simulink library "xps_library"  (Simulink 7.3)
settings: Solver=ode45  SolverMode=SingleTasking  StartTime=0.0  StopTime=10.0  RelTol=1e-3
undefined symbols (not defined in the file): powerpc405, sys_clk, xps_library_software_register_user_data_in
libraries: xbsIndex_r4 x699, simulink x61, casper_library x50, dspsigops x48, xps_library x20, xbsIndex_r3 x2
(part 1 of 9)
settings Model: Creator=hchen05  LastModifiedBy=arccadmin

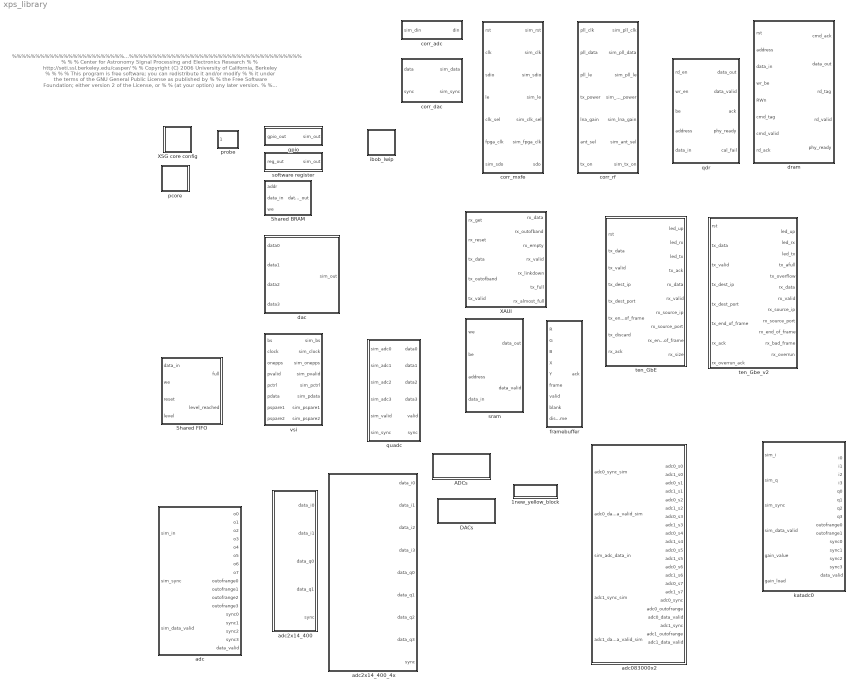
== system xps_library ==
  note: %%%%%%%%%%%%%%%%%%%%%%%%%%%%%%%%%%%%%%%%%%%%%%%%%%%%%%%%%%%%%%%%%%%%%%%%%%%%%%%
      | %                                                                             %
      | %   Center for Astronomy Signal Processing and Electronics Research           %
      | %   http://seti.ssl.berkeley.edu/casper/                                      %
      | %   Copyright (C) 2006 University of California, Berkeley                     %
      | %                                                                             %
      | %   This program is free software; you can redistribute it and/or modify      %
      | %   it under the terms of the GNU General Public License as published by      %
      | %   the Free Software Foundation; either version 2 of the License, or         %
      | %   (at your option) any later version.                                       %
      | %                                                                             %
      | %   This program is distributed in the hope that it will be useful,           %
      | %   but WITHOUT ANY WARRANTY; without even the implied warranty of            %
      | %   MERCHANTABILITY or FITNESS FOR A PARTICULAR PURPOSE.  See the             %
      | %   GNU General Public License for more details.                              %
      | %                                                                             %
      | %   You should have received a copy of the GNU General Public License along   %
      | %   with this program; if not, write to the Free Software Foundation, Inc.,   %
      | %   51 Franklin Street, Fifth Floor, Boston, MA 02110-1301 USA.               %
      | %                                                                             %
      | %%%%%%%%%%%%%%%%%%%%%%%%%%%%%%%%%%%%%%%%%%%%%%%%%%%%%%%%%%%%%%%%%%%%%%%%%%%%%%%
  1new_yellow_block : Subsystem  Tag=xps:block_name
  ADCs : Subsystem
  DACs : Subsystem
  Shared BRAM : Subsystem  Tag=xps:bram  mask{arith_type=Signed  (2's comp), addr_width=11, data_width=32, data_bin_pt=0, init_vals=[1:2^11], sample_rate=1}
      mask prompts: arith_type "Output Data Type"; addr_width "Address width"; data_width "Data Width"; data_bin_pt "Data Binary Point"; init_vals "Initial values (simulation only)"; sample_rate "Sample rate"
      mask init:
      | shared_bram_mask;
      mask StyleString: popup(Unsigned|Signed  (2's comp)),edit,edit,edit,edit,edit
  Shared FIFO : Subsystem  Tag=xps:fifo  mask{io_dir=To Processor, arith_type=Unsigned, data_width=32, data_bin_pt=0, fifo_length=512}
      mask prompts: io_dir "I/O Direction:"; arith_type "Data Type:"; data_width "Data Width:"; data_bin_pt "Data Binary Point:"; fifo_length "Depth:"
      mask init:
      | fifo_mask;
      mask StyleString: popup(From Processor|To Processor),popup(Unsigned|Signed  (2's comp)),popup(4|8|16|32|64|128|256),edit,popup(512|1024|2048|4096|8192|16384|32768|65536)
  XAUI : Subsystem  Tag=xps:xaui  mask(xaui){demux=1, port=ROACH:0, open_phy=on, show_param=off, pre_emph=3, swing=800}
      mask prompts: open_phy "Use KAT open PHY"; show_param "---------------------- Show Implementation Parameters -----------------------------------------------------------------------------------"; pre_emph "Pre-emphasis"; swing "Differential swing"
      mask help: XAUI block for sending and receiving point-to-point, streaming data over the BEE2 and iBOB's CX4 connectors. NOTE: A new version of this block is in development.
      mask init:
      | xaui_mask;
      mask Help: eval('xlWeb([getenv(''MLIB_ROOT''), ''\doc\html\com_xaui\com_xaui.html''])')
      mask StyleString: popup(1|2),popup(iBOB:0|iBOB:1|BEE2_ctrl:0|BEE2_ctrl:1|BEE2_usr:0|BEE2_usr:1|BEE2_usr:2|BEE2_usr:3|CORR:0|ROACH:0|ROACH:1|ROACH:2|ROACH:3),checkbox,checkbox,popup(0|1|2|3),popup(400|500|600|700|800)
      mask CallbackString:
      | |||myname=gcb;
      | if strcmp(get_param(myname, 'show_param'), 'on')
      |     set_param(myname, 'MaskVisibilities', {'on','on','on','on','on','on'});
      | else
      |     set_param(myname, 'MaskVisibilities', {'on','on','on','on','off','off'});
      | end||
  XSG core config : Subsystem  Tag=xps:xsg  mask(xsg core config){hw_sys=iBOB, ibob_linux=off, clk_src=sys_clk, iBOB_clk_src=sys_clk, BEE2_ctrl_clk_src=sys_clk, BEE2_usr_clk_src=sys_clk, ROACH_clk_src=sys_clk, CORR_clk_src=sys_clk, gpio_clk_io_group=iBOB:sma, gpio_clk_bit_index=0, clk_rate=100, sample_period=1, synthesis_tool=XST, mpc_type=powerpc405}
      mask prompts: hw_sys "Hardware Platform"; ibob_linux "Include Linux add-on board support"; clk_src "User IP Clock source"; iBOB_clk_src "User IP Clock source"; BEE2_ctrl_clk_src "User IP Clock Source"; BEE2_usr_clk_src "User IP Clock Source"; ROACH_clk_src "User IP Clock Source"; CORR_clk_src "User IP Clock Source"; gpio_clk_io_group "GPIO Clock Pin I/O group"; gpio_clk_bit_index "GPIO Clock Pin bit index"; clk_rate "User IP Clock Rate (MHz)"; sample_period "Sample Period"; synthesis_tool "Synthesis Tool:"; mpc_type "Processor:"
      mask help:
      | The XSG Core Config block is used to configure the System Generator design
      | for the bee_xps toolflow. Settings here are used to configure the
      | Xilinx System Generator block parameters automatically, and control toolflow
      | script  execution. It needs to be at the top level of all designs being compiled
      | with the bee_xps toolflow.
      mask init:
      | xps_xsg_conf_mask;
      mask Help: eval('xlWeb([getenv(''MLIB_ROOT''), ''\doc\html\sys_xsg_core_config\sys_xsg_core_config.html''])')
      mask StyleString: popup(iBOB|BEE2_ctrl|BEE2_usr|ROACH:sx95t|ROACH:lx110t|CORR),checkbox,edit,popup(sys_clk|sys_clk2x|usr_clk|usr_clk2x|adc0_clk|adc1_clk|dac0_clk|dac1_clk),popup(sys_clk|sys_clk2x|usr_clk|usr_clk2x),popup(sys_clk|sys_clk2x|usr_clk|usr_clk2x),popup(sys_clk|sys_clk2x|arb_clk|aux0_clk|aux0_clk2x|aux1_clk|aux1_clk2x|adc0_clk|adc1_clk|dac0_clk|dac1_clk),popup(sys_clk|sys_clk2x|usr_clk|usr_clk2x),popup(iBOB:gpio0|iBOB:gpio1|iBOB:gpio2|iBOB:gpio3|iBOB:sma|iBOB:zdok0|iBOB:zdok1|iBOB:mdr),edit,edit,edit,popup(Leonardo Spectrum|Synplify|Synplify Pro|XST),edit
      mask CallbackString: xps_xsg_conf_callback;|||xps_xsg_conf_callback;|xps_xsg_conf_callback;|xps_xsg_conf_callback;|xps_xsg_conf_callback;|xps_xsg_conf_callback;||||||
      mask Display: fprintf(['MSSGE\n', hw_sys]);
  adc : Subsystem  Tag=xps:adc  mask(adc){adc_brd=adc0, adc_clk_rate=800, adc_interleave=on, sample_period=1}
      mask prompts: adc_brd "ADC board"; adc_clk_rate "ADC clock rate (MHz)"; adc_interleave "ADC interleave mode"; sample_period "Sample period"
      mask help: The ADC block converts analog inputs to digital outputs. Every clock cycle, the inputs are sampled and digitized to 8 bit binary point numbers in the range of [-1, 1) and are then output by the adc.
      mask init:
      | adc_mask;
      mask Help: eval('xlWeb([getenv(''MLIB_ROOT''), ''\doc\html\sys_adc\sys_adc.html''])')
      mask StyleString: popup(adc0|adc1),edit,checkbox,edit
  adc083000x2 : Subsystem  Tag=xps:adc083000x2  mask(adc_083000x2){use_adc0=on, use_adc1=on, demux_adc=off, clock_sync=on, verbose=off, using_ctrl=on, adc_clk_rate=1000, sample_period=1, bit_width=8}
      mask prompts: use_adc0 "Use ZD0K0?"; use_adc1 "Use ZDOK1?"; demux_adc "Demux ADCs by 2?"; clock_sync "Interleave 2 ADC boards?"; verbose "Verbose Block Creation?"; using_ctrl "Add ports for control registers?"; adc_clk_rate "ADC clock rate (MHz)"; sample_period "Sample Period"; bit_width "Output Bit Width"
      mask help:
      | The ADC block converts analog inputs to digital outputs.
      | Every clock cycle, the inputs are sampled and digitized to
      | 8 bit binary point numbers in the range of [-1, 1).
      |
      | Online block-specific documentation: http://casper.berkeley.edu/wiki/Adc083000
      mask init:
      | adc083000_mask;
      mask Help: eval('xlWeb([getenv(''MLIB_ROOT''), ''\doc\html\sys_adc\sys_adc.html''])')
  adc2x14_400 : Subsystem  Tag=xps:adc2x14_400  mask(ADC board 2xADS5474 Interface Block){adc_brd=0, adc_clk_rate=400}
      mask prompts: adc_brd "ADC Board"; adc_clk_rate "ADC Clock Rate (MHz)"
      mask help: Interface block for the MKID 14-bits 400 MHz ADC board (2xADS5474).
      mask init:
      | adc2x14_400_mask;
      mask StyleString: popup(0|1),edit
  adc2x14_400_4x : Subsystem  Tag=xps:adc2x14_400_4x  mask(2x 14-400 ADC Interface Block){adc_brd=1, adc_clk_rate=400}
      mask prompts: adc_brd "ADC Board"; adc_clk_rate "ADC Clock Rate (MHz)"
      mask help: Interface block for the 14-bits 400 MHz DC board (2xADS5474).
      mask init:
      | adc2x14_400_4x_mask;
      mask StyleString: popup(0|1),edit
  corr_adc : Subsystem  Tag=xps:corr_adc  mask{adc_brd=CORR:adc_i, arith_type=Signed  (2's comp), data_bin_pt=11, reg_clk_phase=0, sample_period=1}
      mask prompts: adc_brd "ADC:"; arith_type "Data type:"; data_bin_pt "Binary point:"; reg_clk_phase "Input sample clock phase:"; sample_period "Sample period:"
      mask init:
      | corr_adc_mask;
      mask StyleString: popup(CORR:adc_i|CORR:adc_q),popup(Unsigned|Signed  (2's comp)),edit,popup(0|90|180|270),edit
  corr_dac : Subsystem  Tag=xps:corr_dac  mask{arith_type=Unsigned, bin_pt=12, reg_clk_phase=0, sample_period=1}
      mask prompts: arith_type "Data Type:"; bin_pt "Data binary point (14-bit data):"; reg_clk_phase "Output sample clock phase:"; sample_period "Sample period:"
      mask init:
      | corr_dac_mask;
      mask StyleString: popup(Boolean|Unsigned|Signed  (2's comp)),edit,popup(0|90|180|270),edit
  corr_mxfe : Subsystem  Tag=xps:corr_mxfe  mask{reg_clk_phase=0, sample_period=1}
      mask prompts: reg_clk_phase "Input sample clock phase:"; sample_period "Sample period:"
      mask init:
      | corr_mxfe_mask;
      mask StyleString: popup(0|90|180|270),edit
  corr_rf : Subsystem  Tag=xps:corr_rf  mask{arith_type=Unsigned, bin_pt=0, sample_period=1}
      mask prompts: arith_type "TX power data type:"; bin_pt "TX power binary point (3-bit data):"; sample_period "Sample period:"
      mask init:
      | corr_rf_mask;
      mask StyleString: popup(Boolean|Unsigned|Signed  (2's comp)),edit,edit
  dac : Subsystem  Tag=xps:dac  mask(dac){dac_brd=iBOB:dac0, dac_clk_rate=800, sample_period=1, show_param=off, invert_clock=off}
      mask prompts: dac_brd "DAC board"; dac_clk_rate "DAC clock rate (MHz)"; sample_period "Sample period"; show_param "---------------------- Show Implementation Parameters -----------------------------------------------------------------------------------"; invert_clock "Invert output clock phase"
      mask help: Interface to SiBeam single Atmel TS86101G2B DAC board. The DAC block converts 4 digital inputs to 1 analog output. The dac runs at 4x FPGA clock frequency, outputting analog converted samples 0 through 3 each FPGA clock cycle.
      mask init:
      | dac_mask;
      mask Help: eval('xlWeb([getenv(''MLIB_ROOT''), ''\doc\html\sys_dac\sys_dac.html''])')
      mask StyleString: popup(iBOB:dac0|iBOB:dac1),edit,edit,checkbox,checkbox
      mask CallbackString:
      | |||myname=gcb;
      | if strcmp(get_param(myname, 'show_param'), 'on')
      |     set_param(myname, 'MaskVisibilities', {'on','on','on','on','on'});
      | else
      |     set_param(myname, 'MaskVisibilities', {'on','on','on','on','off'});
      | end|
  dram : Subsystem  Tag=xps:dram  mask(dram){dimm=1, arith_type=Unsigned, bin_pt=0, ip_clock=200, sample_period=1, bram_fifos=off, disable_tag=off, use_sim=off, ram_depth=18, bank_mgt=off, wide_data=off, half_burst=off, use_sniffer=off}
      mask prompts: arith_type "Data Type"; bin_pt "Data binary point"; ip_clock "Datapath clock rate (MHz)"; sample_period "Sample period"; bram_fifos "Use BRAM FIFOs"; disable_tag "Disable tag FIFO"; use_sim "Simulate DRAM using ModelSim"; ram_depth "Lesser simulation address width"; bank_mgt "Enable bank management"; wide_data "Use wide data bus (288 bits)"; half_burst "Use half-burst"; use_sniffer "Include CPU Interface"
      mask help:
      | Interface to 1GB DDR2 DIMMs on BEE2.
      |
      | To simulate using ModelSim, place a ModelSim block named 'ModelSim' (case-sensitive) in the top level of the design.
      |
      | Commands that are clocked-in are executed with an unknown delay, however, execution order is maintained.
      mask init:
      | dram_mask(gcb, use_sim, wide_data);
      mask Help: eval('xlWeb([getenv(''MLIB_ROOT''), ''\doc\html\sys_dram\sys_dram.html''])')
      mask StyleString: popup(1|2|3|4),popup(Boolean|Unsigned|Signed  (2's comp)),edit,edit,edit,checkbox,checkbox,checkbox,edit,checkbox,checkbox,checkbox,checkbox
      mask CallbackString:
      | |||||||myname=gcb;
      | if strcmp(get_param(myname, 'use_sim'), 'off')
      |     masks = get_param(myname, 'MaskEnables');
      |     masks{9} = 'on';
      |     set_param(myname, 'MaskEnables', masks);
      | else
      |     masks = get_param(myname, 'MaskEnables');
      |     masks{9} = 'off';
      |     set_param(myname, 'MaskEnables', masks);
      | end|||myname=gcb;
      | if strcmp(get_param(myname, 'wide_data'), 'off')
      |     masks = get_param(myname, 'MaskEnables');
      |     masks{12} = 'on';
      |     set_param(myname, 'MaskEnables', masks);
      | else
      |     set_param(myname, 'half_burst', 'off');
      |     masks = get_param(myname, 'MaskEnables');
      |     masks{12} = 'off';
      |     set_param(myname, 'MaskEnables', masks);
      | end||
  framebuffer : Subsystem  Tag=xps:framebuffer  mask(framebuffer){dimm=2, sample_period=1}
      mask prompts: sample_period "Sample period"
      mask help: Interface to Framebuffer.
      mask init:
      | framebuffer_mask;
      mask StyleString: popup(2|3|4),edit
  gpio : Subsystem  Tag=xps:gpio  mask(gpio){io_group=iBOB:led, io_dir=out, arith_type=Boolean, bitwidth=1, bin_pt=0, bit_index=1, sample_period=1, use_single_ended=off, use_ddr=off, reg_iob=on, reg_clk_phase=0, termination=None}
      mask prompts: io_group "I/O group"; io_dir "I/O direction"; arith_type "Data Type"; bitwidth "Data bitwidth"; bin_pt "Data binary point"; bit_index "GPIO bit index"; sample_period "Sample period"; use_single_ended "Use as single-ended"; use_ddr "Use DDR"; reg_iob "Pack register in the pad"; reg_clk_phase "Register clock phase"; termination "Termination method"
      mask help: GPIO interfaces for BEE2, iBOB, ROACH and CORR boards.
      mask init:
      | gpio_mask;
      mask StyleString: popup(iBOB:led|iBOB:dipsw|iBOB:gpio0|iBOB:gpio1|iBOB:gpio2|iBOB:gpio3|iBOB:zdok0|iBOB:zdok1|iBOB:mdr|iBOB:sma|BEE2_ctrl:led|BEE2_ctrl:downlink1|BEE2_ctrl:downlink2|BEE2_ctrl:downlink3|BEE2_ctrl:downlink4|BEE2_usr:led|BEE2_usr:bus_ctrl|BEE2_usr:bus_data|BEE2_usr:uplink|BEE2_usr:leftlink|BEE2_usr:rightlink|ROACH:led|ROACH:gpioa|ROACH:gpioa_oe_n|ROACH:gpiob|ROACH:gpiob_oe_n|ROACH:qsh|ROACH:zdok0|ROACH:zdok1|CORR:four_buttons|CORR:six_buttons|CORR:led|CORR:jumper_driver|CORR:jumper_receiver),popup(in|out),popup(Boolean|Unsigned|Signed  (2's comp)),edit,edit,edit,edit,checkbox,checkbox,checkbox,popup(0|90|180|270),popup(None|Pullup|Pulldown)
      mask CallbackString:
      | if ~isempty(find(strcmp(get_param(gcb, 'io_group'), {'iBOB:zdok0' 'iBOB:zdok1' 'iBOB:mdr' 'ROACH:qsh' 'ROACH:zdok0' 'ROACH:zdok1'})))
      |     set_param(gcb, 'MaskVisibilities', {'on','on','on','on','on','on','on','on','on','on','on','on'});
      | else
      |     set_param(gcb, 'MaskVisibilities', {'on','on','on','on','on','on','on','off','on','on','on','on'});
      | end||||||||if strcmp(get_param(gcb,'use_ddr'),'on')
      |     set_param(gcb,'reg_iob','on');
      |     set_param(gcb,'MaskEnables', {'on' 'on' 'on' 'on' 'on' 'on' 'on' 'on' 'on' 'off' 'on' 'on'});
      | else
      |     set_param(gcb,'MaskEnables', {'on' 'on' 'on' 'on' 'on' 'on' 'on' 'on' 'on' 'on' 'on' 'on'});
      | end|||
  ibob_lwip : Subsystem
      mask Type: ibobethlite
      mask Description: Attaches SRAM0 to the PLB bus and adds LWIP support.
      mask Display: fprintf('IBOB\nLWIP');
  katadc0 : Subsystem  Tag=xps:katadc  mask(adc){adc_brd=adc0, adc_interleave=on, bypass_auto=off, en_gain=on, adc_clk_rate=1000, sample_period=1}
      mask prompts: adc_brd "ADC board"; adc_interleave "ADC interleave mode"; bypass_auto "Bypass auto config"; en_gain "Enable Gain"; adc_clk_rate "ADC clock rate (MHz)"; sample_period "Sample period"
      mask help: The ADC block converts analog inputs to digital outputs. Every clock cycle, the inputs are sampled and digitized to 8 bit binary point numbers in the range of [-1, 1) and are then output by the adc.
      mask init:
      | katadc_mask;
      mask Help: eval('xlWeb([getenv(''MLIB_ROOT''), ''\doc\html\sys_adc\sys_adc.html''])')
      mask StyleString: popup(adc0|adc1),checkbox,checkbox,checkbox,edit,edit
  pcore : Subsystem  Tag=xps:pcore  mask(pcore){pcore_path=customlib/pcores}
      mask prompts: pcore_path "Custom pcores path"
      mask help: Allows insertion of custom EDK pcores not distributed with base systems.
      mask Display: fprintf('PCORE');
  probe : Subsystem  Tag=xps:probe  mask{ila_number=0, match_type=basic, match_counter_width=8, capture_depth=512, arith_type=Boolean, bitwidth=1, bin_pt=0}
      mask prompts: ila_number "Chipscope ILA number"; match_type "Match Unit Type"; match_counter_width "Match counter width"; capture_depth "Probe capture depth"; arith_type "Data type"; bitwidth "Data bit width"; bin_pt "Data binary point"
      mask init:
      | probe_mask;
      mask StyleString: popup(0|1|2|3|4|5|6|7|8|9|10|11|12|13|14),popup(basic|basic with edges|extended|extended with edges|range|range with edges),popup(0|8|16|24|32),popup(512|1024|2048|4096|8192|16384),popup(Boolean|Unsigned|Signed  (2's comp)),edit,edit
  qdr : Subsystem  Tag=xps:qdr  mask(qdr){which_qdr=qdr0, qdr_awidth=12, use_sniffer=off}
      mask prompts: which_qdr "QDR Chip"; qdr_awidth "Simulation QDR address width"; use_sniffer "Include CPU Interface"
      mask help: Interface to the QDR II SRAM device on ROACH
      mask init:
      | qdr_mask(gcb);
      mask StyleString: popup(qdr0|qdr1),edit,checkbox
  quadc : Subsystem  Tag=xps:quadc  mask(CASPER QuADC Interface Block){adc_brd=0, adc_clk_rate=200}
      mask prompts: adc_brd "ADC Board"; adc_clk_rate "ADC Clock Rate (MHz)"
      mask help: Interface block for the CASPER Quad ADC board (ADC4x250-8).
      mask init:
      | quadc_mask;
      mask StyleString: popup(0|1),edit
  software register : Subsystem  Tag=xps:sw_reg  mask{io_dir=To Processor, arith_type=Unsigned, bitwidth=32, bin_pt=0, sample_period=1, gw_name=xps_library_software_register_user_data_in}
      mask prompts: io_dir "I/O direction"; arith_type "Data Type"; bitwidth "Data bitwidth"; bin_pt "Data binary point"; sample_period "Sample period"; gw_name "Mask Parameter 6:"
      mask init:
      | register_mask;
      mask StyleString: popup(From Processor|To Processor),popup(Unsigned|Signed  (2's comp)),edit,edit,edit,edit
  sram : Subsystem  Tag=xps:sram  mask(sram){sram=1, arith_type=Unsigned, bin_pt=0, sample_period=1, use_sim=on}
      mask prompts: arith_type "Data Type"; bin_pt "Data binary point (bitwidth is 36)"; sample_period "Sample period"; use_sim "Simulate SRAM using ModelSim"
      mask help:
      | Interface to CY7C1370DV25 36x512k SRAMs on IBOB.
      |
      | To simulate using ModelSim, place a ModelSim block named 'ModelSim' (case-sensitive) in the top level of the design.
      |
      | The sram block represents a 36x512k SRAM chip on the IBOB. It stores 36-bit words and requires 19 bits to access its address space.
      mask init:
      | sram_mask;
      mask Help: eval('xlWeb([getenv(''MLIB_ROOT''), ''\doc\html\sys_sram\sys_sram.html''])')
      mask StyleString: popup(0|1),popup(Boolean|Unsigned|Signed  (2's comp)),edit,edit,checkbox
  ten_GbE : Subsystem  Tag=xps:tengbe  mask(ten_GbE){port=BEE2_ctrl:0, mac_lite=off, open_phy=off, show_param=off, pre_emph=3, swing=800, fab_en=off, fab_mac=0, fab_ip=0, fab_udp=0, fab_gate=0}
      mask prompts: mac_lite "Use light-weight MAC: Warning --> it DOES NOT check any CRC on receive"; open_phy "Use KAT open XAUI PHY"; show_param "---------------------- Show Implementation Parameters -----------------------------------------------------------------------------------"; pre_emph "Pre-emphasis"; swing "Differential swing"; fab_en "Enable fabric on startup"; fab_mac "Fabric MAC Address"; fab_ip "Fabric IP Address"; fab_udp "Fabric UDP Port"; fab_gate "Fabric Gateway"
      mask help: This block sends and receives UDP frames (packets). It accepts a 64 bit wide data stream with user-determined frame breaks. The data stream is wrapped in a UDP frame for transmission. Incoming UDP packets are unwrapped and the data presented as a 64 bit wide stream.
      mask init:
      | tengbe_mask;
      mask Help: eval('xlWeb([getenv(''MLIB_ROOT''), ''\doc\html\com_ten_GbE\com_ten_GbE.html''])')
      mask StyleString: popup(BEE2_ctrl:0|BEE2_ctrl:1|BEE2_usr:0|BEE2_usr:1|BEE2_usr:2|BEE2_usr:3|iBOB:0|iBOB:1|ROACH:0|ROACH:1|ROACH:2|ROACH:3),checkbox,checkbox,checkbox,popup(0|1|2|3),popup(400|500|600|700|800),checkbox,edit,edit,edit,edit
      mask CallbackString:
      | |||myname=gcb;
      | if strcmp(get_param(myname, 'show_param'), 'on')
      |     set_param(myname, 'MaskVisibilities', {'on','on','on','on','on', 'on','on','on','on','on', 'on',});
      | else
      |     set_param(myname, 'MaskVisibilities', {'on','on','on','on','off','off','off','off','off','off','off'});
      | end|||||||
  ten_Gbe_v2 : Subsystem  Tag=xps:tengbe_v2  mask(ten_GbE_v2){port=0, rx_dist_ram=on, large_frames=off, show_param=on, pre_emph=3, swing=800, fab_en=on, fab_mac=hex2dec('123456780000'), fab_ip=192*(2^24) + 168*(2^16) + 5*(2^8) + 20*(2^0), fab_udp=10000, fab_gate=1, cpu_rx_en=on, cpu_tx_en=on}
      mask prompts: rx_dist_ram "Shallow RX Fifo (Beware overruns!)"; large_frames "Enable Large TX Frames (8k+512)"; show_param "---------------------- Show Implementation Parameters -----------------------------------------------------------------------------------"; pre_emph "Pre-emphasis"; swing "Differential swing"; fab_en "Enable fabric on startup"; fab_mac "Fabric MAC Address"; fab_ip "Fabric IP Address"; fab_udp "Fabric UDP Port"; fab_gate "Fabric Gateway"; cpu_rx_en "Enable CPU RX"; cpu_tx_en "Enable CPU TX"
      mask help: This block sends and receives UDP frames (packets). It accepts a 64 bit wide data stream with user-determined frame breaks. The data stream is wrapped in a UDP frame for transmission. Incoming UDP packets are unwrapped and the data presented as a 64 bit wide stream.
      mask init:
      | tengbe_v2_mask;
      mask StyleString: popup(0|1|2|3),checkbox,checkbox,checkbox,popup(0|1|2|3),popup(400|500|600|700|800),checkbox,edit,edit,edit,edit,checkbox,checkbox
      mask CallbackString:
      | |||myname=gcb;
      | if strcmp(get_param(myname, 'show_param'), 'on')
      |     set_param(myname, 'MaskVisibilities', {'on', 'on', 'on','on','on','on','on','on','on','on','on','on','on'});
      | else
      |     set_param(myname, 'MaskVisibilities', {'on', 'on', 'on','on','off','off','off','off','off','off','off','off','off'});
      | end|||||||||
  vsi : Subsystem  Tag=xps:vsi  mask(vsi){connector=MDR, arith_type=Unsigned, bin_pt=0, sample_period=1}
      mask prompts: arith_type "Data Type"; bin_pt "Data binary point (bitwidth is 32)"; sample_period "Sample period"
      mask help: Interface to MDR-80 connector on IBOB as configured for VLBI Standard Interface.
      mask init:
      | vsi_mask;
      mask StyleString: popup(MDR|ZDOK 1),popup(Boolean|Unsigned|Signed  (2's comp)),edit,edit

== system xps_library/1new_yellow_block ==

== system xps_library/ADCs ==
  adc083000_ctrl : Subsystem  Tag=xps:adc083000_ctrl  mask(adc083000_ctrl){}
      mask init:
      | adc083000_ctrl_mask;
  adc2x14_400 : xps_library/adc2x14_400  Tag=xps:adc2x14_400  SystemSampleTime=-1  adc_brd=0  adc_clk_rate=400
  adc2x14_400_4x : xps_library/adc2x14_400_4x  Tag=xps:adc2x14_400_4x  SystemSampleTime=-1  adc_brd=1  adc_clk_rate=400
  adc_mkid : Subsystem  Tag=xps:adc_mkid  mask(MKID ADC Interface Block){adc_brd=1, adc_clk_rate=512}
      mask prompts: adc_brd "ADC Board"; adc_clk_rate "ADC Clock Rate (MHz)"
      mask help: Interface block for the MKID 12-bits 550 MHz ADC board (2xADS54RF63).
      mask init:
      | adc_mkid_mask;
      mask StyleString: popup(0|1),edit
  adc_sim : Subsystem  mask(adc_sim){nStreams=8, bit_width=8}
      mask prompts: nStreams "Number of Output Streams"; bit_width "Sample Bit Width"
      mask help:
      | This block simulates the behavior of a demuxed ADC, which takes
      | as input a waveform and returns digital samples in parallel at
      | a slower rate.
      |
      | This block is used to simulate the behavior
      mask init:
      | adc_sim_init(gcb, ...
      |     'nStreams', nStreams, ...
      |     'bit_width', bit_width);
  conv : Subsystem  mask{bit_width=8}
      mask prompts: bit_width "Bit Width"
      mask help:
      | Converts an (8-bit) unsigned number to 2's complement.
      | This block should eventually be able to handle arbitrary
      | width inputs.
      mask init:
      | % set_param([gcb, '/Slice1'], 'nbits', num2str(bit_width-1));
      | % set_param([gcb, '/Reinterpret'], 'bin_pt', num2str(bit_width-1));
  of1 : Subsystem  mask(of){bit_num=0, n_adc_bits=8}
      mask prompts: bit_num "Bit index of overflow detection bus:"; n_adc_bits "Number of bits in ADC"
      mask help: 1-cycle overflow detector for an n-bit ADC outputs (simulation only)
  of_detect_bus : Subsystem  mask(of_detect_bus){nStreams=8, bit_width=8}
      mask prompts: nStreams "Number of Streams"; bit_width "Bit Width"
      mask init:
      | of_detect_bus_init(gcb, ...
      |     'nStreams', nStreams, ...
      |     'bit_width', bit_width);

== system xps_library/DACs ==
  dac_mkid : Subsystem  Tag=xps:dac_mkid  mask(MKID DAC Interface Block){dac_brd=0, dac_clk_rate=512, sample_period=1}
      mask prompts: dac_brd "DAC board"; dac_clk_rate "DAC external clock rate (MHz)"; sample_period "Sample period"
      mask help: Interface block for the MKID 16-bits DAC board (2xDAC5681)
      mask init:
      | dac_mkid_mask;
      mask StyleString: popup(0|1),edit,edit

== system xps_library/Shared BRAM ==
  addr : Inport  OutDataType=sfix(16)  OutScaling=2^0
  data_in : Inport  Port=2  OutDataType=sfix(16)  OutScaling=2^0
  we : Inport  Port=3  OutDataType=sfix(16)  OutScaling=2^0
  convert_addr : xbsIndex_r4/Convert  arith_type=Unsigned  n_bits=addr_width  bin_pt=0  quantization=Truncate  overflow=Wrap  latency=0  dbl_ovrd=off  pipeline=off  block_type=convert
      settings: xl_area=[0, 0, 0, 0, 0, 0, 0]
  convert_din : xbsIndex_r4/Convert  arith_type="Signed  (2's comp)"  n_bits=data_width  bin_pt=data_bin_pt  quantization=Truncate  overflow=Wrap  latency=0  dbl_ovrd=off  pipeline=off  block_type=convert
      settings: xl_area=[0, 0, 0, 0, 0, 0, 0]
  convert_we : xbsIndex_r4/Convert  arith_type=Unsigned  n_bits=1  bin_pt=0  quantization=Truncate  overflow=Wrap  latency=0  dbl_ovrd=off  pipeline=off  block_type=convert
      settings: xl_area=[0, 0, 0, 0, 0, 0, 0]
  mem : Subsystem
  xps_library_Shared_BRAM_addr : xbsIndex_r4/Gateway Out  hdl_port=on  timing_constraint=None  locs_specified=off  LOCs={'A5','B9','A9','C1','A3','G6','E9','A6','A7','A8','B8','B1','B3','D9','B5','B4','B6','C2'}  block_type=gatewayout
      settings: infoedit="Gateway out block.  Converts Xilinx fixed point inputs into ouputs of type Simulink integer, double, or fixed point.<P><P>Hardware notes:  In hardware these blocks become top level output ports or are discarded, depending on how they are configured."  xl_area=[0, 0, 0, 0, 0, 0, 0]  sginterface={'Nallatech'=>{'xdspkit'=>{'non_memory_mapped_port'=>'uprev_Shared_BRAM_addr'}},'Xilinx'=>{'jtaghwcosim'=>{'non_memory_mapped_port'=>'uprev_Shared_BRAM_addr'},'xdspkit'=>{'non_memory_mapped_port'=>'uprev_Shared_BRAM_addr'}}}
  xps_library_Shared_BRAM_data_in : xbsIndex_r4/Gateway Out  hdl_port=on  timing_constraint=None  locs_specified=off  LOCs={'B21','B22','A22','B23','B19','C19','A20','A21','A23','B24','A24','A25','E18','D18','C18','B18'}  block_type=gatewayout
      settings: infoedit="Gateway out block.  Converts Xilinx fixed point inputs into ouputs of type Simulink integer, double, or fixed point.<P><P>Hardware notes:  In hardware these blocks become top level output ports or are discarded, depending on how they are configured."  xl_area=[0, 0, 0, 0, 0, 0, 0]  sginterface={'Nallatech'=>{'xdspkit'=>{'non_memory_mapped_port'=>'uprev_Shared_BRAM_data_in'}},'Xilinx'=>{'jtaghwcosim'=>{'non_memory_mapped_port'=>'uprev_Shared_BRAM_data_in'},'xdspkit'=>{'non_memory_mapped_port'=>'uprev_Shared_BRAM_data_in'}}}
  xps_library_Shared_BRAM_data_out : xbsIndex_r4/Gateway In  arith_type="Signed  (2's comp)"  n_bits=data_width  bin_pt=data_bin_pt  quantization=Truncate  overflow=Wrap  period=sample_rate  dbl_ovrd=off  timing_constraint=None  locs_specified=off  LOCs={}  block_type=gatewayin
      settings: infoedit="Gateway in block.  Converts inputs of type Simulink integer, double and fixed point to  Xilinx fixed point type.<P><P>Hardware notes:  In hardware these blocks become top level input ports."  xl_area=[0, 0, 0, 0, 0, 0, 0]
  xps_library_Shared_BRAM_we : xbsIndex_r4/Gateway Out  hdl_port=on  timing_constraint=None  locs_specified=off  LOCs={'A14'}  block_type=gatewayout
      settings: infoedit="Gateway out block.  Converts Xilinx fixed point inputs into ouputs of type Simulink integer, double, or fixed point.<P><P>Hardware notes:  In hardware these blocks become top level output ports or are discarded, depending on how they are configured."  xl_area=[0, 0, 0, 0, 0, 0, 0]
  data_out : Outport  OutDataType=sfix(16)  OutScaling=2^0
  wires:
  mem/1(Out1) -> xps_library_Shared_BRAM_data_out/1
  data_in/1 -> convert_din/1
  xps_library_Shared_BRAM_data_out/1 -> data_out/1
  addr/1 -> convert_addr/1
  we/1 -> convert_we/1
  convert_addr/1 -> xps_library_Shared_BRAM_addr/1
  convert_we/1 -> xps_library_Shared_BRAM_we/1
  convert_din/1 -> xps_library_Shared_BRAM_data_in/1
  xps_library_Shared_BRAM_addr/1 -> mem/1(In1)
  xps_library_Shared_BRAM_data_in/1 -> mem/2(In2)
  xps_library_Shared_BRAM_we/1 -> mem/3(In3)

== system xps_library/Shared FIFO ==
  data_in : Inport  OutDataType=sfix(16)  OutScaling=2^0
  we : Inport  Port=2  OutDataType=sfix(16)  OutScaling=2^0
  reset : Inport  Port=3  OutDataType=sfix(16)  OutScaling=2^0
  level : Inport  Port=4  OutDataType=sfix(16)  OutScaling=2^0
  convert_untitled_Shared_FIFO_user_data_in : xbsIndex_r4/Convert  arith_type=Unsigned  n_bits=32  bin_pt=0  quantization=Truncate  overflow=Wrap  latency=0  dbl_ovrd=off  pipeline=off  block_type=convert
  convert_untitled_Shared_FIFO_user_level : xbsIndex_r4/Convert  arith_type=Unsigned  n_bits=16  bin_pt=0  quantization=Truncate  overflow=Wrap  latency=0  dbl_ovrd=off  pipeline=off  block_type=convert
  convert_untitled_Shared_FIFO_user_reset : xbsIndex_r4/Convert  arith_type=Unsigned  n_bits=1  bin_pt=0  quantization=Truncate  overflow=Wrap  latency=0  dbl_ovrd=off  pipeline=off  block_type=convert
  convert_untitled_Shared_FIFO_user_we : xbsIndex_r4/Convert  arith_type=Unsigned  n_bits=1  bin_pt=0  quantization=Truncate  overflow=Wrap  latency=0  dbl_ovrd=off  pipeline=off  block_type=convert
  untitled_Shared_FIFO_user_data_in : xbsIndex_r4/Gateway Out  hdl_port=on  timing_constraint=None  locs_specified=off  LOCs={}  block_type=gatewayout
      settings: infoedit="Gateway out block.  Converts Xilinx fixed point inputs into ouputs of type Simulink integer, double, or fixed point.<P><P>Hardware notes:  In hardware these blocks become top level output ports or are discarded, depending on how they are configured."
  untitled_Shared_FIFO_user_full : xbsIndex_r4/Gateway In  arith_type=Unsigned  n_bits=1  bin_pt=0  quantization="Round  (unbiased: +/- Inf)"  overflow=Saturate  period=1  dbl_ovrd=off  timing_constraint=None  locs_specified=off  LOCs={}  block_type=gatewayin
      settings: infoedit="Gateway in block.  Converts inputs of type Simulink integer, double and fixed point to  Xilinx fixed point type.<P><P>Hardware notes:  In hardware these blocks become top level input ports."
  untitled_Shared_FIFO_user_full_const : Constant  Value=0  OutDataType=sfix(16)  OutScaling=2^0
  untitled_Shared_FIFO_user_level : xbsIndex_r4/Gateway Out  hdl_port=on  timing_constraint=None  locs_specified=off  LOCs={}  block_type=gatewayout
      settings: infoedit="Gateway out block.  Converts Xilinx fixed point inputs into ouputs of type Simulink integer, double, or fixed point.<P><P>Hardware notes:  In hardware these blocks become top level output ports or are discarded, depending on how they are configured."
  untitled_Shared_FIFO_user_level_reached : xbsIndex_r4/Gateway In  arith_type=Unsigned  n_bits=1  bin_pt=0  quantization="Round  (unbiased: +/- Inf)"  overflow=Saturate  period=1  dbl_ovrd=off  timing_constraint=None  locs_specified=off  LOCs={}  block_type=gatewayin
      settings: infoedit="Gateway in block.  Converts inputs of type Simulink integer, double and fixed point to  Xilinx fixed point type.<P><P>Hardware notes:  In hardware these blocks become top level input ports."
  untitled_Shared_FIFO_user_level_reached_const : Constant  Value=0  OutDataType=sfix(16)  OutScaling=2^0
  untitled_Shared_FIFO_user_reset : xbsIndex_r4/Gateway Out  hdl_port=on  timing_constraint=None  locs_specified=off  LOCs={}  block_type=gatewayout
      settings: infoedit="Gateway out block.  Converts Xilinx fixed point inputs into ouputs of type Simulink integer, double, or fixed point.<P><P>Hardware notes:  In hardware these blocks become top level output ports or are discarded, depending on how they are configured."
  untitled_Shared_FIFO_user_we : xbsIndex_r4/Gateway Out  hdl_port=on  timing_constraint=None  locs_specified=off  LOCs={}  block_type=gatewayout
      settings: infoedit="Gateway out block.  Converts Xilinx fixed point inputs into ouputs of type Simulink integer, double, or fixed point.<P><P>Hardware notes:  In hardware these blocks become top level output ports or are discarded, depending on how they are configured."
  full : Outport  OutDataType=sfix(16)  OutScaling=2^0
  level_reached : Outport  Port=2  OutDataType=sfix(16)  OutScaling=2^0
  wires:
  untitled_Shared_FIFO_user_level_reached_const/1 -> untitled_Shared_FIFO_user_level_reached/1
  untitled_Shared_FIFO_user_level_reached/1 -> level_reached/1
  untitled_Shared_FIFO_user_full_const/1 -> untitled_Shared_FIFO_user_full/1
  untitled_Shared_FIFO_user_full/1 -> full/1
  convert_untitled_Shared_FIFO_user_level/1 -> untitled_Shared_FIFO_user_level/1
  level/1 -> convert_untitled_Shared_FIFO_user_level/1
  convert_untitled_Shared_FIFO_user_reset/1 -> untitled_Shared_FIFO_user_reset/1
  reset/1 -> convert_untitled_Shared_FIFO_user_reset/1
  convert_untitled_Shared_FIFO_user_we/1 -> untitled_Shared_FIFO_user_we/1
  we/1 -> convert_untitled_Shared_FIFO_user_we/1
  convert_untitled_Shared_FIFO_user_data_in/1 -> untitled_Shared_FIFO_user_data_in/1
  data_in/1 -> convert_untitled_Shared_FIFO_user_data_in/1

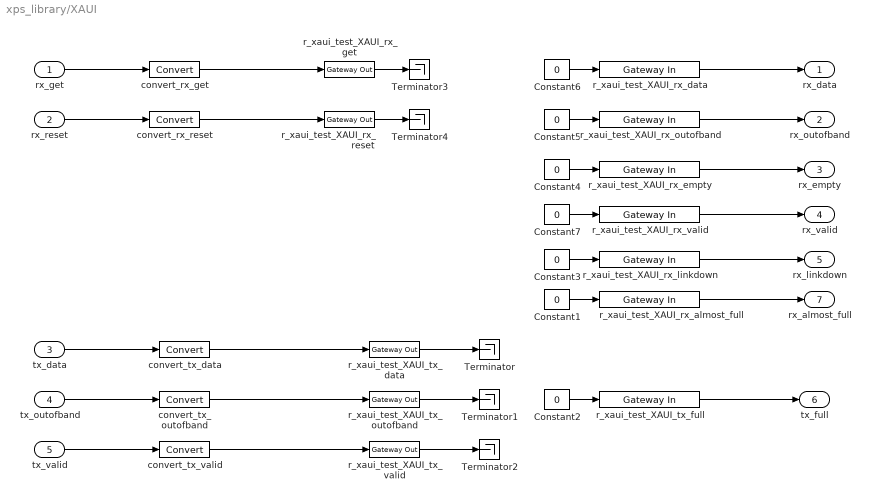
== system xps_library/XAUI ==
  rx_get : Inport  OutDataType=sfix(16)  OutScaling=2^0
  rx_reset : Inport  Port=2  OutDataType=sfix(16)  OutScaling=2^0
  tx_data : Inport  Port=3  OutDataType=sfix(16)  OutScaling=2^0
  tx_outofband : Inport  Port=4  OutDataType=sfix(16)  OutScaling=2^0
  tx_valid : Inport  Port=5  OutDataType=sfix(16)  OutScaling=2^0
  Constant{1..7} (7 alike) : Constant  Value=0  OutDataType=sfix(16)  OutScaling=2^0
  Terminator{,1..4} (5 alike) : Terminator
  convert_rx_get : xbsIndex_r4/Convert  arith_type=Boolean  n_bits=64  bin_pt=0  quantization=Truncate  overflow=Wrap  latency=0  dbl_ovrd=off  pipeline=off  block_type=convert
      settings: xl_area=[0, 0, 0, 0, 0, 0, 0]
  convert_rx_reset : xbsIndex_r4/Convert  arith_type=Boolean  n_bits=1  bin_pt=0  quantization=Truncate  overflow=Wrap  latency=0  dbl_ovrd=off  pipeline=off  block_type=convert
      settings: xl_area=[0, 0, 0, 0, 0, 0, 0]
  convert_tx_data : xbsIndex_r4/Convert  arith_type=Unsigned  n_bits=64  bin_pt=0  quantization=Truncate  overflow=Wrap  latency=0  dbl_ovrd=off  pipeline=off  block_type=convert
      settings: xl_area=[0, 0, 0, 0, 0, 0, 0]
  convert_tx_outofband : xbsIndex_r4/Convert  arith_type=Unsigned  n_bits=8  bin_pt=0  quantization=Truncate  overflow=Wrap  latency=0  dbl_ovrd=off  pipeline=off  block_type=convert
      settings: xl_area=[0, 0, 0, 0, 0, 0, 0]
  convert_tx_valid : xbsIndex_r4/Convert  arith_type=Boolean  n_bits=1  bin_pt=0  quantization=Truncate  overflow=Wrap  latency=0  dbl_ovrd=off  pipeline=off  block_type=convert
      settings: xl_area=[0, 0, 0, 0, 0, 0, 0]
  r_xaui_test_XAUI_rx_almost_full : xbsIndex_r4/Gateway In  arith_type=Boolean  n_bits=1  bin_pt=0  quantization=Truncate  overflow=Wrap  period=1  dbl_ovrd=off  timing_constraint=None  locs_specified=off  LOCs={}  block_type=gatewayin
      settings: infoedit="Gateway in block.  Converts inputs of type Simulink integer, double and fixed point to  Xilinx fixed point type.<P><P>Hardware notes:  In hardware these blocks become top level input ports."  xl_area=[0, 0, 0, 0, 0, 0, 0]
  r_xaui_test_XAUI_rx_data : xbsIndex_r4/Gateway In  arith_type=Unsigned  n_bits=64  bin_pt=0  quantization=Truncate  overflow=Wrap  period=1  dbl_ovrd=off  timing_constraint=None  locs_specified=off  LOCs={}  block_type=gatewayin
      settings: infoedit="Gateway in block.  Converts inputs of type Simulink integer, double and fixed point to  Xilinx fixed point type.<P><P>Hardware notes:  In hardware these blocks become top level input ports."  xl_area=[0, 0, 0, 0, 0, 0, 0]
  r_xaui_test_XAUI_rx_empty : xbsIndex_r4/Gateway In  arith_type=Boolean  n_bits=1  bin_pt=0  quantization=Truncate  overflow=Wrap  period=1  dbl_ovrd=off  timing_constraint=None  locs_specified=off  LOCs={}  block_type=gatewayin
      settings: infoedit="Gateway in block.  Converts inputs of type Simulink integer, double and fixed point to  Xilinx fixed point type.<P><P>Hardware notes:  In hardware these blocks become top level input ports."  xl_area=[0, 0, 0, 0, 0, 0, 0]
  r_xaui_test_XAUI_rx_get : xbsIndex_r4/Gateway Out  hdl_port=on  timing_constraint=None  locs_specified=off  LOCs={}  block_type=gatewayout
      settings: infoedit="Gateway out block.  Converts Xilinx fixed point inputs into ouputs of type Simulink integer, double, or fixed point.<P><P>Hardware notes:  In hardware these blocks become top level output ports or are discarded, depending on how they are configured."  xl_area=[0, 0, 0, 0, 0, 0, 0]
  r_xaui_test_XAUI_rx_linkdown : xbsIndex_r4/Gateway In  arith_type=Boolean  n_bits=1  bin_pt=0  quantization=Truncate  overflow=Wrap  period=1  dbl_ovrd=off  timing_constraint=None  locs_specified=off  LOCs={}  block_type=gatewayin
      settings: infoedit="Gateway in block.  Converts inputs of type Simulink integer, double and fixed point to  Xilinx fixed point type.<P><P>Hardware notes:  In hardware these blocks become top level input ports."  xl_area=[0, 0, 0, 0, 0, 0, 0]
  r_xaui_test_XAUI_rx_outofband : xbsIndex_r4/Gateway In  arith_type=Unsigned  n_bits=8  bin_pt=0  quantization=Truncate  overflow=Wrap  period=1  dbl_ovrd=off  timing_constraint=None  locs_specified=off  LOCs={}  block_type=gatewayin
      settings: infoedit="Gateway in block.  Converts inputs of type Simulink integer, double and fixed point to  Xilinx fixed point type.<P><P>Hardware notes:  In hardware these blocks become top level input ports."  xl_area=[0, 0, 0, 0, 0, 0, 0]
  r_xaui_test_XAUI_rx_reset : xbsIndex_r4/Gateway Out  hdl_port=on  timing_constraint=None  locs_specified=off  LOCs={}  block_type=gatewayout
      settings: infoedit="Gateway out block.  Converts Xilinx fixed point inputs into ouputs of type Simulink integer, double, or fixed point.<P><P>Hardware notes:  In hardware these blocks become top level output ports or are discarded, depending on how they are configured."  xl_area=[0, 0, 0, 0, 0, 0, 0]
  r_xaui_test_XAUI_rx_valid : xbsIndex_r4/Gateway In  arith_type=Boolean  n_bits=1  bin_pt=0  quantization=Truncate  overflow=Wrap  period=1  dbl_ovrd=off  timing_constraint=None  locs_specified=off  LOCs={}  block_type=gatewayin
      settings: infoedit="Gateway in block.  Converts inputs of type Simulink integer, double and fixed point to  Xilinx fixed point type.<P><P>Hardware notes:  In hardware these blocks become top level input ports."  xl_area=[0, 0, 0, 0, 0, 0, 0]
  r_xaui_test_XAUI_tx_data : xbsIndex_r4/Gateway Out  hdl_port=on  timing_constraint=None  locs_specified=off  LOCs={}  block_type=gatewayout
      settings: infoedit="Gateway out block.  Converts Xilinx fixed point inputs into ouputs of type Simulink integer, double, or fixed point.<P><P>Hardware notes:  In hardware these blocks become top level output ports or are discarded, depending on how they are configured."  xl_area=[0, 0, 0, 0, 0, 0, 0]
  r_xaui_test_XAUI_tx_full : xbsIndex_r4/Gateway In  arith_type=Boolean  n_bits=1  bin_pt=0  quantization=Truncate  overflow=Wrap  period=1  dbl_ovrd=off  timing_constraint=None  locs_specified=off  LOCs={}  block_type=gatewayin
      settings: infoedit="Gateway in block.  Converts inputs of type Simulink integer, double and fixed point to  Xilinx fixed point type.<P><P>Hardware notes:  In hardware these blocks become top level input ports."  xl_area=[0, 0, 0, 0, 0, 0, 0]
  r_xaui_test_XAUI_tx_outofband : xbsIndex_r4/Gateway Out  hdl_port=on  timing_constraint=None  locs_specified=off  LOCs={}  block_type=gatewayout
      settings: infoedit="Gateway out block.  Converts Xilinx fixed point inputs into ouputs of type Simulink integer, double, or fixed point.<P><P>Hardware notes:  In hardware these blocks become top level output ports or are discarded, depending on how they are configured."  xl_area=[0, 0, 0, 0, 0, 0, 0]
  r_xaui_test_XAUI_tx_valid : xbsIndex_r4/Gateway Out  hdl_port=on  timing_constraint=None  locs_specified=off  LOCs={}  block_type=gatewayout
      settings: infoedit="Gateway out block.  Converts Xilinx fixed point inputs into ouputs of type Simulink integer, double, or fixed point.<P><P>Hardware notes:  In hardware these blocks become top level output ports or are discarded, depending on how they are configured."  xl_area=[0, 0, 0, 0, 0, 0, 0]
  rx_data : Outport  OutDataType=sfix(16)  OutScaling=2^0
  rx_outofband : Outport  Port=2  OutDataType=sfix(16)  OutScaling=2^0
  rx_empty : Outport  Port=3  OutDataType=sfix(16)  OutScaling=2^0
  rx_valid : Outport  Port=4  OutDataType=sfix(16)  OutScaling=2^0
  rx_linkdown : Outport  Port=5  OutDataType=sfix(16)  OutScaling=2^0
  tx_full : Outport  Port=6  OutDataType=sfix(16)  OutScaling=2^0
  rx_almost_full : Outport  Port=7  OutDataType=sfix(16)  OutScaling=2^0
  wires:
  Constant1/1 -> r_xaui_test_XAUI_rx_almost_full/1
  r_xaui_test_XAUI_rx_almost_full/1 -> rx_almost_full/1
  r_xaui_test_XAUI_rx_valid/1 -> rx_valid/1
  Constant7/1 -> r_xaui_test_XAUI_rx_valid/1
  r_xaui_test_XAUI_rx_reset/1 -> Terminator4/1
  r_xaui_test_XAUI_rx_get/1 -> Terminator3/1
  Constant6/1 -> r_xaui_test_XAUI_rx_data/1
  Constant5/1 -> r_xaui_test_XAUI_rx_outofband/1
  Constant4/1 -> r_xaui_test_XAUI_rx_empty/1
  Constant3/1 -> r_xaui_test_XAUI_rx_linkdown/1
  Constant2/1 -> r_xaui_test_XAUI_tx_full/1
  r_xaui_test_XAUI_tx_valid/1 -> Terminator2/1
  r_xaui_test_XAUI_tx_outofband/1 -> Terminator1/1
  r_xaui_test_XAUI_tx_data/1 -> Terminator/1
  r_xaui_test_XAUI_tx_full/1 -> tx_full/1
  convert_tx_valid/1 -> r_xaui_test_XAUI_tx_valid/1
  tx_valid/1 -> convert_tx_valid/1
  convert_tx_outofband/1 -> r_xaui_test_XAUI_tx_outofband/1
  tx_outofband/1 -> convert_tx_outofband/1
  convert_tx_data/1 -> r_xaui_test_XAUI_tx_data/1
  tx_data/1 -> convert_tx_data/1
  r_xaui_test_XAUI_rx_linkdown/1 -> rx_linkdown/1
  r_xaui_test_XAUI_rx_empty/1 -> rx_empty/1
  r_xaui_test_XAUI_rx_outofband/1 -> rx_outofband/1
  r_xaui_test_XAUI_rx_data/1 -> rx_data/1
  convert_rx_reset/1 -> r_xaui_test_XAUI_rx_reset/1
  rx_reset/1 -> convert_rx_reset/1
  convert_rx_get/1 -> r_xaui_test_XAUI_rx_get/1
  rx_get/1 -> convert_rx_get/1

== system xps_library/XSG core config ==
